simulink model "practicad1"  (R2015a)
settings: Solver=ode3  StartTime=0.0  StopTime=10.0  FixedStep=1  RelTol=1e-3
settings Model: Creator=sala3  LastModifiedBy=Jesus

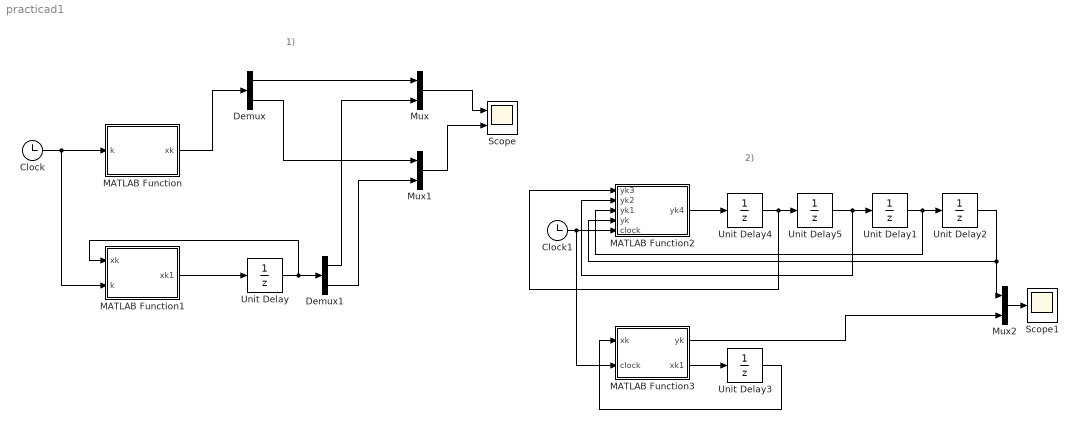
== system practicad1 ==
  note: 2)
  note: 1)
  Clock : Clock
  Clock1 : Clock
  Demux : Demux  Outputs=2
  Demux1 : Demux  Outputs=2
  MATLAB Function : MATLAB Function  TreatAsAtomicUnit=on
  MATLAB Function1 : MATLAB Function  TreatAsAtomicUnit=on
  MATLAB Function2 : MATLAB Function  TreatAsAtomicUnit=on
  MATLAB Function3 : MATLAB Function  TreatAsAtomicUnit=on
  Mux : Mux  Inputs=2
  Mux1 : Mux  Inputs=2
  Mux2 : Mux  Inputs=2
  Scope : Scope  NumInputPorts=2
      settings: YMin=-5~-5  YMax=5~5
  Scope1 : Scope
  Unit Delay : UnitDelay  InitialCondition=[-1;4]  SampleTime=-1
  Unit Delay1 : UnitDelay  InitialCondition=298  SampleTime=-1
  Unit Delay2 : UnitDelay  InitialCondition=-5  SampleTime=-1
  Unit Delay3 : UnitDelay  InitialCondition=[1;2;-1;-3;]  SampleTime=-1
  Unit Delay4 : UnitDelay  InitialCondition=49231  SampleTime=-1
  Unit Delay5 : UnitDelay  InitialCondition=4992.8  SampleTime=-1
  wires:
  Clock/1 -> MATLAB Function1/2(k), MATLAB Function/1(k)
  MATLAB Function/1(xk) -> Demux/1
  MATLAB Function1/1(xk1) -> Unit Delay/1
  Unit Delay/1 -> Demux1/1, MATLAB Function1/1(xk)
  Mux/1 -> Scope/1
  Demux/1 -> Mux/1
  Demux1/1 -> Mux/2
  Mux1/1 -> Scope/2
  Demux/2 -> Mux1/1
  Demux1/2 -> Mux1/2
  Unit Delay4/1 -> MATLAB Function2/1(yk3), Unit Delay5/1
  Unit Delay5/1 -> MATLAB Function2/2(yk2), Unit Delay1/1
  Clock1/1 -> MATLAB Function3/2(clock), MATLAB Function2/5(clock)
  MATLAB Function2/1(yk4) -> Unit Delay4/1
  Unit Delay1/1 -> MATLAB Function2/3(yk1), Unit Delay2/1
  Unit Delay2/1 -> Mux2/1, MATLAB Function2/4(yk)
  MATLAB Function3/2(xk1) -> Unit Delay3/1
  Unit Delay3/1 -> MATLAB Function3/1(xk)
  MATLAB Function3/1(yk) -> Mux2/2
  Mux2/1 -> Scope1/1

== matlab function practicad1/MATLAB Function1 ==
  data: xk1 output; xk input; k input
function xk1  = fcn(xk,k)
%#codegen
A=[0 1;-1/10 7/10];
B=[3/10;-1/10];
u=-5*cos(k);
xk1=A*xk+B*u;

== matlab function practicad1/MATLAB Function ==
  data: xk output; k input
function xk  = fcn(k)
%#codegen
 xk=[(207*sin(k - 1) + 723*sin(k + 1) + 1551*sin(k - 2) - 90*sin(k + 2) - 930*sin(k - 3) - 1461*sin(k) + 25504*(1/2)^k*sin(1) - 14920*(1/2)^k*sin(2) + 2000*(1/2)^k*sin(3) - 27700*(1/5)^k*sin(1) + 17485*(1/5)^k*sin(2) - 3050*(1/5)^k*sin(3))/(1680*sin(1) - 924*sin(2) + 120*sin(3));
        (291*sin(k - 1) - 201*sin(k + 1) - 237*sin(k - 2) + 30*sin(k + 2) - 90*sin(k - 3) + 207*sin(k) + 12752*(1/2)^k*sin(1) - 7460*(1/2)^k*sin(2) + 1000*(1/2)^k*sin(3) - 5540*(1/5)^k*sin(1) + 3497*(1/5)^k*sin(2) - 610*(1/5)^k*sin(3))/(1680*sin(1) - 924*sin(2) + 120*sin(3))];

== matlab function practicad1/MATLAB Function2 ==
  data: yk3 input; yk2 input; yk1 input; yk input; clock input; yk4 output
function yk4 = fcn(yk3,yk2,yk1,yk,clock)
%#codegen
k=clock;
uk3=sin(k+3);
uk2=sin(k+2);
yk4=16*yk3-96*yk2+256*yk1-256*yk+uk3+2*uk2;

== matlab function practicad1/MATLAB Function3 ==
  data: yk output; xk input; xk1 output; clock input
function [yk,xk1] = fcn(xk,clock)
%#codegen
uk=clock;
A=[0 1 0 0;0 0 1 0;0 0 0 1;-256 256 -96 16];
B=[0 0 0 1]';
C=[0 0 2 1];
xk1= A*xk + B*uk;
yk=C*xk;
